simulink model "PSOFuzzyPar"  (R2024b)
settings: Solver=VariableStepAuto  StartTime=0.0  StopTime=20  RelTol=1e-3
undefined symbols (not defined in the file or in its folder): Kd, Kp
settings Model: Creator=david  LastModifiedBy=david

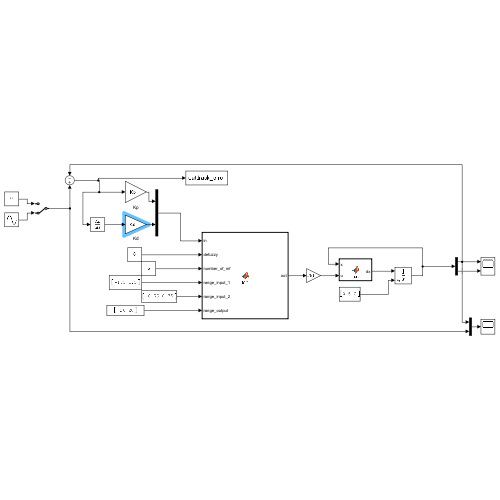
[thumbnail: Simulink's stored preview of the top-level diagram]
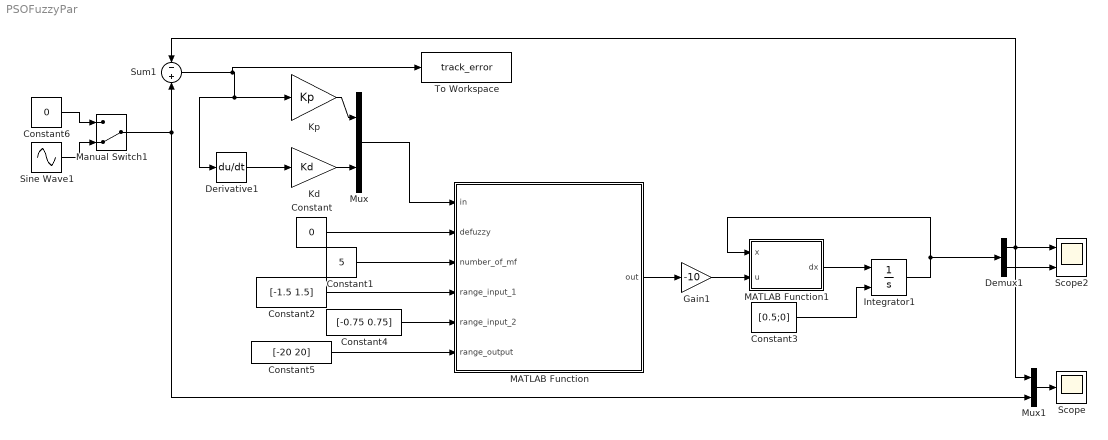
== system PSOFuzzyPar ==
  Constant : Constant  Value=0
  Constant1 : Constant  Value=5
  Constant2 : Constant  Value=[-1.5 1.5]
  Constant3 : Constant  Value=[0.5;0]
  Constant4 : Constant  Value=[-0.75 0.75]
  Constant5 : Constant  Value=[-20 20]
  Constant6 : Constant  Value=0
  Demux1 : Demux  Outputs=2
  Derivative1 : Derivative
  Gain1 : Gain  Gain=-10
  Integrator1 : Integrator  InitialConditionSource=external
  Kd : Gain  Gain=Kd
  Kp : Gain  Gain=Kp
  MATLAB Function : MATLAB Function  TreatAsAtomicUnit=on
  MATLAB Function1 : MATLAB Function  TreatAsAtomicUnit=on
  Manual Switch1 : ManualSwitch  CurrentSetting=0
  Mux : Mux  Inputs=2
  Mux1 : Mux  Inputs=2
  Scope : Scope
  Scope2 : Scope  NumInputPorts=2
  Sine Wave1 : Sin  Amplitude=.25  Frequency=4  SampleTime=0
  Sum1 : Sum  Inputs=-|+
  To Workspace : ToWorkspace  VariableName=track_error  SampleTime=-1
  wires:
  Integrator1/1 -> MATLAB Function1/1(x), Demux1/1
  Demux1/1 -> Scope2/1, Mux1/1, Sum1/1
  Demux1/2 -> Scope2/2
  Constant3/1 -> Integrator1/2
  Gain1/1 -> MATLAB Function1/2(u)
  MATLAB Function/1(out) -> Gain1/1
  MATLAB Function1/1(dx) -> Integrator1/1
  Constant/1 -> MATLAB Function/2(defuzzy)
  Constant1/1 -> MATLAB Function/3(number_of_mf)
  Constant2/1 -> MATLAB Function/4(range_input_1)
  Constant4/1 -> MATLAB Function/5(range_input_2)
  Constant5/1 -> MATLAB Function/6(range_output)
  Sine Wave1/1 -> Manual Switch1/2
  Manual Switch1/1 -> Sum1/2, Mux1/2
  Sum1/1 -> To Workspace/1, Derivative1/1, Kp/1
  Constant6/1 -> Manual Switch1/1
  Derivative1/1 -> Kd/1
  Kd/1 -> Mux/2
  Kp/1 -> Mux/1
  Mux/1 -> MATLAB Function/1(in)
  Mux1/1 -> Scope/1

== matlab function PSOFuzzyPar/MATLAB Function1 ==
  data: x input; dx output; u input
function dx  = fcn(x,u)

m = 1;
k=2;
b=0.2;


x1 = x(1);
x2 = x(2);
dx1 = -(k/m)*x2 + (1/m)*u;
dx2 = x1 - (b/m)*x2;
dx = [dx1;dx2];

y = u;

== matlab function PSOFuzzyPar/MATLAB Function ==
  data: in input; out output; defuzzy input; number_of_mf input; range_input_1 input; range_input_2 input; range_output input
function out = fcn(in, defuzzy, number_of_mf, range_input_1, range_input_2, range_output)
% in: [error, d_error]
% defuzzy: 0 = COG, 1 = CA
% range_input_1/2: [min, max]
% range_output: [min, max]

% === 1. Preparar divisiones ===
div1 = linspace(range_input_1(1), range_input_1(2), number_of_mf); % error
div2 = linspace(range_input_2(1), range_input_2(2), number_of_mf); % d_error
div_out = linspace(range_output(1), range_output(2), number_of_mf); % salida

% === 2. Calcular membresías de entrada ===
mu_e = compute_memberships(in(1), div1);
mu_de = compute_memberships(in(2), div2);

% === 3. Definir FAM ===
FAM = zeros(number_of_mf, number_of_mf);
middle_val = (number_of_mf + 1) / 2;
middle_ij = middle_val*2;
for i = 1:number_of_mf
    for j = 1:number_of_mf
        FAM(i,j) = middle_val + middle_ij - (i + j);
        if FAM(i,j) > number_of_mf 
            FAM(i,j) = number_of_mf;
        end
        if FAM(i,j) < 1
            FAM(i,j) = 1;
        end
    end
end

% === 4. Activaciones de reglas ===
rule_heights = zeros(number_of_mf,number_of_mf);
for i = 1:number_of_mf
    for j = 1:number_of_mf
        out_idx = FAM(i,j);
        h = min(mu_e(i), mu_de(j));
        rule_heights(i,j) = h;
    end
end

% Max activación por salida
mu_out = zeros(1,number_of_mf);
for k = 1:number_of_mf
    mu_out(k) = max(rule_heights(FAM==k));
end

% === 5. Defuzzificación ===
if defuzzy == 0
    % COG
    num = 0; den = 0;
    step = div_out(2)-div_out(1);
    base = 2*step; % base total de cada triángulo
    for k = 1:number_of_mf
        h = mu_out(k);
        if h > 0
            % Base efectiva (triángulo truncado horizontalmente)
            top_base = (1-h)*base;
            A = h*(base+top_base)/2; % área del trapecio
            num = num + A*div_out(k);
            den = den + A;
        end
    end
    if den == 0
        out = div_out(3); % centro
    else
        out = num/den;
    end
else
    % CA (Weighted Average by heights)
    num = sum(mu_out .* div_out);
    den = sum(mu_out);
    if den == 0
        out = div_out(3);
    else
        out = num/den;
    end
end
end

% === Membresías ===
function mu = compute_memberships(x, div)
% Devuelve vector de 5 membresías triangulares
n = length(div);
mu = zeros(1,n);

if x <= div(1)
    mu(1) = 1; return
elseif x >= div(end)
    mu(end) = 1; return
end

for i = 1:n-1
    x1 = div(i); x2 = div(i+1);
    if x >= x1 && x <= x2
        mu(i) = (x2 - x)/(x2 - x1);
        mu(i+1) = (x - x1)/(x2 - x1);
        return
    end
end
end
